simulink model "SimulacionControlSysNoLineal_Simplificado_Qube"  (R2017a)
settings: Solver=ode4  StartTime=0.0  StopTime=10  FixedStep=0.002  RelTol=1e-3  EnableMultiTasking=on
values from neighbouring files (symbols this model uses):
  betaP = 0.0005    [ParametrosModeloNOlinealPendulo.m]
  betaR = 0.0015    [ParametrosModeloNOlinealPendulo.m]
  g = 9.8    [ParametrosModeloNOlinealPendulo.m]
  Jb = Mb*Lb^2/12    (= 5.71979166667e-05)    [ParametrosModeloNOlinealPendulo.m]
  Jp = Mp*(Lcm*2)^2/12    (= 3.3282e-05)    [ParametrosModeloNOlinealPendulo.m]
  K = Keq*inv(P)    [ParametrosModeloNOlinealPendulo.m]
  kc = dcgain(salBra)    [ParametrosModeloNOlinealPendulo.m]
  km = 0.042    [ParametrosModeloNOlinealPendulo.m]
  Lb = 0.085    [ParametrosModeloNOlinealPendulo.m]
  Lcm = 0.129/2    (= 0.0645)    [ParametrosModeloNOlinealPendulo.m]
  Mp = 0.024    [ParametrosModeloNOlinealPendulo.m]
  Rm = 8.4    [ParametrosModeloNOlinealPendulo.m]
libraries: simulink_extras x3, simulink x2
settings Model: Creator=Alejandra  LastModifiedBy=sebastian.jimenez1
settings DataIOCC: LimitDataPoints=on  SaveFormat=Array
settings OptimizationCC: LifeSpan=inf
settings DebuggingCC: SFUnexpectedBacktrackingDiag=warning  SFNoUnconditionalDefaultTransitionDiag=warning  SFExecutionAtInitializationDiag=none
settings HardwareCC: ProdBitPerPointer=32  ProdBitPerSizeT=32  ProdBitPerPtrDiffT=32  ProdLargestAtomicFloat=None  ProdIntDivRoundTo=Undefined  ProdEndianess=Unspecified  ProdWordSize=32  ProdHWDeviceType=32-bit Generic
settings ModelReferenceCC: PropagateSignalLabelsOutOfModel=off
settings GRTTargetCC: TargetLangStandard=C89/C90 (ANSI)  GeneratePreprocessorConditionals=Disable all
settings ConfigComp: CovMetricSettings=dw  CovHtmlReporting=on  CovSaveCumulativeToWorkspaceVar=on  CovSaveSingleToWorkspaceVar=on  CovExternalEMLEnable=off

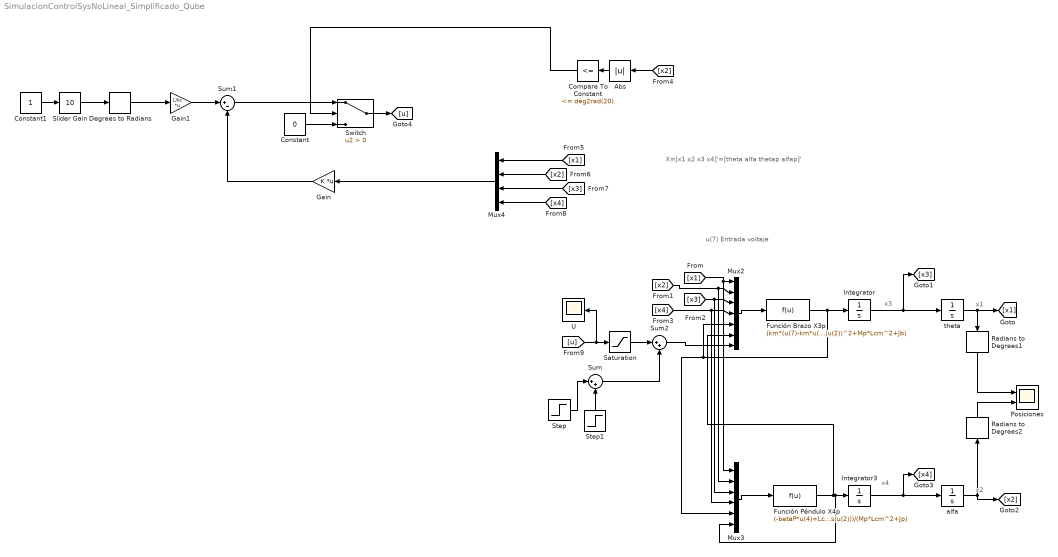
== system SimulacionControlSysNoLineal_Simplificado_Qube ==
  note: u(7) Entrada voltaje
  note: x4
  note: x3
  note: x2
  note: x1
  note: X=[x1 x2 x3 x4]'=[theta alfa thetap alfap]'
  Abs : Abs
  Compare To Constant : simulink/Logic and Bit Operations/Compare To Constant  relop=<=  const=deg2rad(20)  OutDataTypeStr=boolean
  Constant : Constant  Value=0
  Constant1 : Constant
  Degrees to Radians : simulink_extras/Transformations/Degrees to Radians
  Función Brazo X3p : Fcn  Expr=(km*(u(7)-km*u(3))/(Rm)-betaR*u(3)+(Lb*Lcm*Mp*u(4)^2*sin(u(2)))-Lb*Lcm*Mp*u(6)*cos(u(2))-2*Lcm^2*Mp*u(3)*u(4)*cos(u(2))*sin(u(2)))/(Mp*Lb^2-Mp*Lcm^2*cos(u(2))^2+Mp*Lcm^2+Jb)
  Función Péndulo X4p : Fcn  Expr=(-betaP*u(4)+Lcm^2*Mp*Lcm^2*cos(u(2))*sin(u(2))+Lcm*Mp*g*sin(u(2))-Lb*Lcm*Mp*u(5)*cos(u(2)))/(Mp*Lcm^2+Jp)
  Gain : Gain  Gain=K  Multiplication=Matrix(K*u)
  Gain1 : Gain  Gain=1/kc  Multiplication=Matrix(K*u)
  Integrator : Integrator
  Integrator3 : Integrator
  Mux2 : Mux  Inputs=7
  Mux3 : Mux  Inputs=6
  Mux4 : Mux
  Posiciones : Scope  NumInputPorts=2
  Radians to Degrees1 : simulink_extras/Transformations/Radians to Degrees
  Radians to Degrees2 : simulink_extras/Transformations/Radians to Degrees
  Saturation : Saturate  UpperLimit=10  LowerLimit=-10
  Slider Gain : simulink/Math Operations/Slider Gain  gain=10  low=-90  high=90
  Step : Step  Time=1.5  After=5  SampleTime=0
  Step1 : Step  After=-5  SampleTime=0
  Sum : Sum  Inputs=|++
  Sum1 : Sum  Inputs=|+-
  Sum2 : Sum  Inputs=|++
  Switch : Switch  Criteria=u2 > Threshold
  U : Scope
  alfa : Integrator
  theta : Integrator
  wires:
  Integrator3/1 -> [x4], alfa/1
  Integrator/1 -> [x3], theta/1
  alfa/1 -> [x2], Radians to Degrees2/1
  Función Brazo X3p/1 -> Mux3/5, Mux2/5, Integrator/1
  Mux2/1 -> Función Brazo X3p/1
  Función Péndulo X4p/1 -> Mux2/6, Mux3/6, Integrator3/1
  theta/1 -> Radians to Degrees1/1, [x1]
  [x1] -> Mux3/1, Mux2/1
  [x2] -> Mux3/2, Mux2/2
  [x3] -> Mux3/3, Mux2/3
  [x4] -> Mux3/4, Mux2/4
  Mux3/1 -> Función Péndulo X4p/1
  Gain1/1 -> Sum1/1
  Gain/1 -> Sum1/2
  Slider Gain/1 -> Degrees to Radians/1
  Constant/1 -> Switch/3
  Constant1/1 -> Slider Gain/1
  Degrees to Radians/1 -> Gain1/1
  Abs/1 -> Compare To Constant/1
  [x2] -> Abs/1
  Compare To Constant/1 -> Switch/2
  [x2] -> Mux4/2
  [x1] -> Mux4/1
  [x3] -> Mux4/3
  [x4] -> Mux4/4
  Mux4/1 -> Gain/1
  Switch/1 -> [u]
  [u] -> U/1, Saturation/1
  Step/1 -> Sum/1
  Step1/1 -> Sum/2
  Sum/1 -> Sum2/2
  Sum2/1 -> Mux2/7
  Radians to Degrees1/1 -> Posiciones/1
  Radians to Degrees2/1 -> Posiciones/2
  Saturation/1 -> Sum2/1
  Sum1/1 -> Switch/1
